simulink model "FIR_Filter"  (R2020a)
settings: Solver=FixedStepAuto  StartTime=0.0  StopTime=10.0  FixedStep=1  RelTol=1e-3
settings Model: Creator=Admin  LastModifiedBy=Admin
settings DataIOCC: SaveOutput=off  SaveTime=off

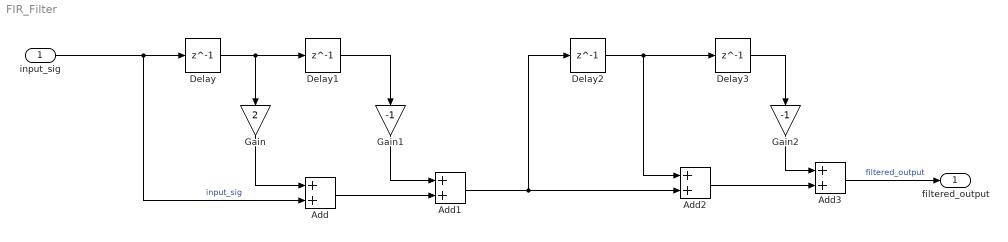
== system FIR_Filter ==
  input_sig : Inport  OutDataTypeStr=double  PortDimensions=[1 1]  SampleTime=[1,0]
  Add{,1..3} (4 alike) : Sum
  Delay{,1..3} (4 alike) : Delay  DelayLength=1
  Gain : Gain  Gain=2
  Gain1 : Gain  Gain=-1
  Gain2 : Gain  Gain=-1
  filtered_output : Outport  OutDataTypeStr=double  PortDimensions=[1 1]  SampleTime=[1,0]
  wires:
  Gain1/1 -> Add1/1
  input_sig/1 -> Delay/1, Add/2  "input_sig"
  Gain/1 -> Add/1
  Delay/1 -> Delay1/1, Gain/1
  Gain2/1 -> Add3/1
  Add1/1 -> Delay2/1, Add2/2
  Delay2/1 -> Add2/1, Delay3/1
  Delay3/1 -> Gain2/1
  Add/1 -> Add1/2
  Add3/1 -> filtered_output/1  "filtered_output"
  Add2/1 -> Add3/2
  Delay1/1 -> Gain1/1
